simulink model "pendulum"  (Simulink 7.1)
settings: Solver=FixedStepDiscrete  StartTime=0.0  StopTime=10.0  FixedStep=1e-3  RelTol=1e-3
libraries: MBDynCom x3
settings Model: Creator=masarati  LastModifiedBy=marco  ExtModeAutoUpdateStatusClock=off
settings DataIOCC: SignalLoggingName=sigsOut
settings DebuggingCC: SaveWithParameterizedLinksMsg=none  SignalResolutionControl=TryResolveAllWithWarning  SolverPrmCheckMsg=none  MultiTaskDSMMsg=warning  MultiTaskCondExecSysMsg=none  StrictBusMsg=None
settings HardwareCC: TargetUnknown=on
settings RTWCC: IncludeERTFirstTime=on
settings GRTTargetCC: TargetFcnLib=ansi_tfl_tmw.mat

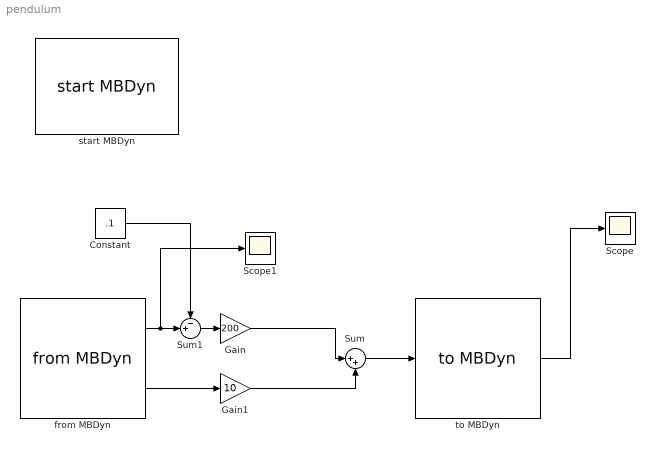
== system pendulum ==
  Constant : Constant  Value=.1  OutDataType=sfix(16)  OutScaling=2^0
  Gain : Gain  Gain=200  ParameterDataType=sfix(16)  ParameterScaling=2^0  OutDataType=sfix(16)  OutScaling=2^0  SaturateOnIntegerOverflow=on  OutDataTypeStr=Inherit: Same as input  ParamDataTypeStr=Inherit: Same as input
  Gain1 : Gain  Gain=10  ParameterDataType=sfix(16)  ParameterScaling=2^0  OutDataType=sfix(16)  OutScaling=2^0  SaturateOnIntegerOverflow=on  OutDataTypeStr=Inherit: Same as input  ParamDataTypeStr=Inherit: Same as input
  Scope : Scope
      settings: YMin=-20  YMax=12.5
  Scope1 : Scope
      settings: YMin=0  YMax=0.175
  Sum : Sum  Inputs=|++  OutDataType=sfix(16)  OutScaling=2^0  SaturateOnIntegerOverflow=on
  Sum1 : Sum  Inputs=-+|  OutDataType=sfix(16)  OutScaling=2^0  SaturateOnIntegerOverflow=on
  from MBDyn : MBDynCom/from MBDyn  Priority=0  RTAI_flag=off  Socket_flag=on  mbdtask='MBDTSK'  mbx='MBXINN'  net=on  node='127.0.0.1'  port=10011  path='tmp/mbdyn.pendulum.out.sock'  N_chan=2  Tc=1e-3
  start MBDyn : MBDynCom/start MBDyn  enable_path=on  mbdyn_path='./mbdyn.sh'  input_file='examples/pendulum'  enable_out=on  output_file='tmp/pendulum_controlled'  verbose=off  pedantic=off
  to MBDyn : MBDynCom/to MBDyn  Priority=0  RTAI_flag=off  Socket_flag=on  mbdtask='MBDTSK'  mbx='MBXOUT'  net=on  node='127.0.0.1'  port=8005  path='/tmp/mbdyn.pendulum.in.sock'  N_chan=1  Tc=1e-3
  wires:
  from MBDyn/2 -> Gain1/1
  Gain1/1 -> Sum/2
  Gain/1 -> Sum/1
  Sum/1 -> to MBDyn/1
  from MBDyn/1 -> Sum1/2, Scope1/1
  Sum1/1 -> Gain/1
  Constant/1 -> Sum1/1
  to MBDyn/1 -> Scope/1
